simulink model "Discrete_rudder_system_disc_copy1"  (R2017a)
settings: Solver=VariableStepAuto  StartTime=0.0  StopTime=10.0  RelTol=1e-3
values from neighbouring files (symbols this model uses):
  A = [-4.65E-06	0.0001701	-0.0002836	0	0	0	-2.56E-06	-7.97E-06	3.61E-06 ... (first row only)    [surfaces_setup_test.m]
  B = [-7.98E-09	7.83E-09	1.68E-09	2.75E-10 ... (first row only)    [surfaces_setup_test.m]
  X0 = [w_B_BE_ini;Theta_ini;Vbbe_int]    [surfaces_setup_test.m]
libraries: simulink x1
settings Model: Creator=Jiaoran Wang  LastModifiedBy=Jiaoran Wang

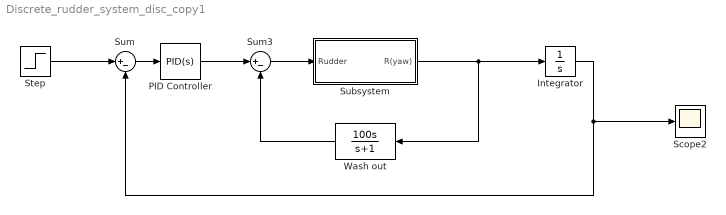
== system Discrete_rudder_system_disc_copy1 ==
  Integrator : Integrator
  PID Controller : simulink/Continuous/PID Controller  Controller=PID  TimeDomain=Continuous-time  SampleTime=-1  IntegratorMethod=Forward Euler  FilterMethod=Forward Euler  Form=Parallel  UseFilter=on  ControllerParametersSource=internal  P=1000  I=0  D=1  N=100  InitialConditionSource=internal  InitialConditionForIntegrator=0  InitialConditionForFilter=0  ExternalReset=none  LimitOutput=off  UpperSaturationLimit=inf  LowerSaturationLimit=-inf  LinearizeAsGain=on  AntiWindupMode=none  Kb=1  TrackingMode=off  Kt=1  PParamMin=[]  PParamMax=[]  IParamMin=[]  IParamMax=[]  DParamMin=[]  DParamMax=[]  NParamMin=[]  NParamMax=[]  KbParamMin=[]  KbParamMax=[]  KtParamMin=[]  KtParamMax=[]  POutMin=[]  POutMax=[]  IOutMin=[]  IOutMax=[]  DOutMin=[]  DOutMax=[]  NOutMin=[]  NOutMax=[]  KbOutMin=[]  KbOutMax=[]  KtOutMin=[]  KtOutMax=[]  IntegratorOutMin=[]  IntegratorOutMax=[]  FilterOutMin=[]  FilterOutMax=[]  SumOutMin=[]  SumOutMax=[]  SumI1OutMin=[]  SumI1OutMax=[]  SumI2OutMin=[]  SumI2OutMax=[]  SumI3OutMin=[]  SumI3OutMax=[]  SumDOutMin=[]  SumDOutMax=[]  SaturationOutMin=[]  SaturationOutMax=[]  IntegratorContinuousStateAttributes=''  IntegratorStateMustResolveToSignalObject=off  IntegratorRTWStateStorageClass=Auto  FilterContinuousStateAttributes=''  FilterStateMustResolveToSignalObject=off  FilterRTWStateStorageClass=Auto  DifferentiatorICPrevScaledInput=0  DifferentiatorOutMin=[]  DifferentiatorOutMax=[]  InitialConditionSetting=State (most efficient)
  Scope2 : Scope
  Step : Step  After=-20000  SampleTime=0
  Subsystem : Subsystem
  Sum : Sum  Inputs=|+-
  Sum3 : Sum  Inputs=|+-
  Wash out : TransferFcn  Numerator=[100 0]  Denominator=[1 1]
  wires:
  Subsystem/1(R(yaw)) -> Wash out/1, Integrator/1
  Sum3/1 -> Subsystem/1(Rudder)
  Sum/1 -> PID Controller/1
  PID Controller/1 -> Sum3/1
  Wash out/1 -> Sum3/2
  Integrator/1 -> Sum/2, Scope2/1
  Step/1 -> Sum/1

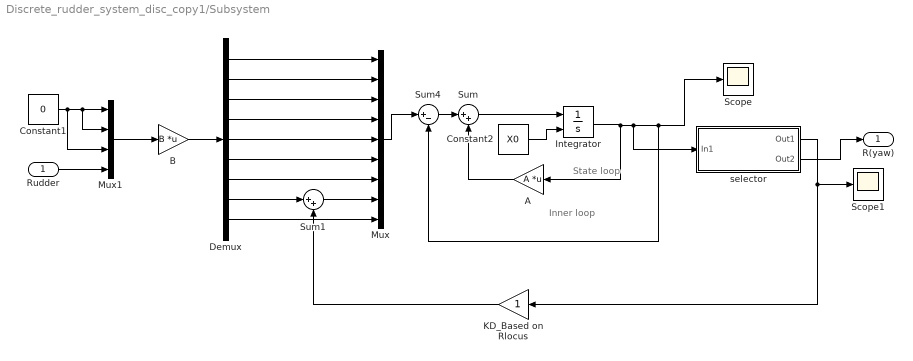
== system Discrete_rudder_system_disc_copy1/Subsystem ==
  note: Inner loop
  note: State loop
  Rudder : Inport
  A : Gain  Gain=A  Multiplication=Matrix(K*u)
  B : Gain  Gain=B  Multiplication=Matrix(K*u)
  Constant1 : Constant  Value=0
  Constant2 : Constant  Value=X0
  Demux : Demux  Outputs=9
  Integrator : Integrator  InitialConditionSource=external
  KD_Based on Rlocus : Gain
  Mux : Mux  Inputs=9
  Mux1 : Mux
  Scope : Scope
  Scope1 : Scope
  Sum : Sum  Inputs=|++
  Sum1 : Sum  Inputs=|++
  Sum4 : Sum  Inputs=|+-
  selector : Subsystem
  R(yaw) : Outport
  wires:
  Demux/7 -> Mux/7
  Demux/6 -> Mux/6
  Constant2/1 -> Integrator/2
  Demux/3 -> Mux/3
  Sum/1 -> Integrator/1
  selector/1(Out1) -> Scope1/1, KD_Based on Rlocus/1
  B/1 -> Demux/1
  Demux/2 -> Mux/2
  Demux/4 -> Mux/4
  Demux/9 -> Mux/9
  Integrator/1 -> selector/1(In1), Sum4/2, Scope/1, A/1
  Sum4/1 -> Sum/1
  A/1 -> Sum/2
  Demux/5 -> Mux/5
  Demux/1 -> Mux/1
  Mux/1 -> Sum4/1
  Mux1/1 -> B/1
  Constant1/1 -> Mux1/3, Mux1/2, Mux1/1
  Rudder/1 -> Mux1/4
  selector/2(Out2) -> R(yaw)/1
  Demux/8 -> Sum1/1
  KD_Based on Rlocus/1 -> Sum1/2
  Sum1/1 -> Mux/8

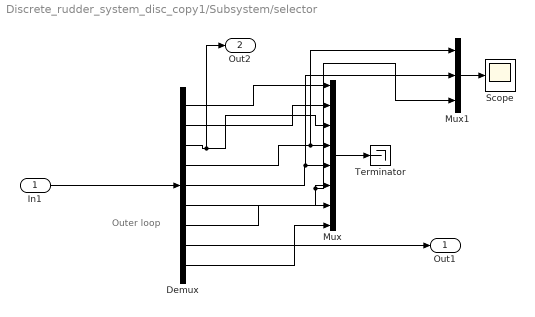
== system Discrete_rudder_system_disc_copy1/Subsystem/selector ==
  note: Outer loop
  In1 : Inport
  Demux : Demux  Outputs=9
  Mux : Mux  Inputs=8
  Mux1 : Mux  Inputs=3
  Scope : Scope
  Terminator : Terminator
  Out1 : Outport
  Out2 : Outport  Port=2
  wires:
  Demux/5 -> Mux1/2, Mux/5
  Demux/1 -> Mux/1
  Demux/3 -> Out2/1, Mux/3
  Demux/2 -> Mux/2
  In1/1 -> Demux/1
  Demux/4 -> Mux1/1, Mux/4
  Demux/6 -> Mux1/3, Mux/6
  Demux/7 -> Mux/7
  Mux/1 -> Terminator/1
  Demux/8 -> Out1/1
  Demux/9 -> Mux/8
  Mux1/1 -> Scope/1
